simulink library "gravity_lib"  (Simulink 6.6)
libraries: simulink x1
settings Model: Creator=amurch  LastModifiedBy=cox  ExtModeAutoUpdateStatusClock=off

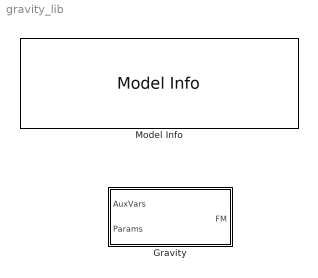
== system gravity_lib ==
  Gravity : Subsystem
  Model Info : simulink/Model-Wide Utilities/Model Info  SystemSampleTime=-1  InitialBlockCM=None  BlockCM=None  Frame=on  DisplayStringWithTags=|  HorizontalTextAlignment=Center  LeftAlignmentValue=0.5  SourceBlockDiagram=gravity_lib  TagMaxNumber=20
      | Gravity Model Library
      | %<ModelVersion>
      | Las modified by %<LastModifiedBy> on %<LastModificationDate>

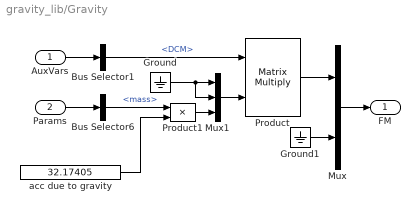
== system gravity_lib/Gravity ==
  AuxVars : Inport
  Params : Inport  Port=2
  Bus Selector1 : BusSelector  OutputSignals=DCM
  Bus Selector6 : BusSelector  OutputSignals=mass
  Ground : Ground
  Ground1 : Ground
  Mux : Mux  Inputs=[3 3]
  Mux1 : Mux  Inputs=3
  Product : Product  Multiplication=Matrix(*)  RndMeth=Zero
  Product1 : Product  RndMeth=Zero
  acc due to gravity : Constant  Value=32.17405
  FM : Outport
  wires:
  Bus Selector6/1 -> Product1/1  "<mass>"
  Bus Selector1/1 -> Product/1  "<DCM>"
  AuxVars/1 -> Bus Selector1/1
  Params/1 -> Bus Selector6/1
  Product/1 -> Mux/1
  Mux/1 -> FM/1
  Mux1/1 -> Product/2
  Ground/1 -> Mux1/1, Mux1/2
  Product1/1 -> Mux1/3
  Ground1/1 -> Mux/2
  acc due to gravity/1 -> Product1/2
